simulink model "Child_fuzzy"  (R2023a)
settings: Solver=FixedStepAuto  StartTime=0.0  StopTime=inf  RelTol=1e-3
undefined symbols (not defined in the file): Data_Display, Data_Display1, Data_Display2, Data_Display3, Data_Display4, Data_Display5, Proj
libraries: androiduilib x9, androidaudiovideolib x4, androidcommunicationlib x4, androidsensorlib x3, fuzblock x2
settings Model: Creator=hp  LastModifiedBy=hp
settings OptimizationCC: EnhancedBackFolding=on  PassReuseOutputArgsAs=Individual arguments  ZeroExternalMemoryAtStartup=off  ZeroInternalMemoryAtStartup=off  MaxStackSize=64  OptimizeBlockOrder=speed  DifferentSizesBufferReuse=on  OptimizationCustomize=off  EfficientTunableParamExpr=on
settings DebuggingCC: ParameterTunabilityLossMsg=error
settings HardwareCC: ProdBitPerPointer=32  ProdBitPerSizeT=32  ProdBitPerPtrDiffT=32  ProdLargestAtomicInteger=Long  ProdLargestAtomicFloat=Double  ProdWordSize=32  ProdHWDeviceType=ARM Compatible->ARM Cortex
settings SFSimCC: MATLABDynamicMemAlloc=off
settings RTWCC: Description=Embedded Coder  SystemTargetFile=ert.tlc  HardwareBoard=Android Device  TLCOptions="-aInlineSetEventsForThisBaseRateFcn=TLC_FALSE -aSuppressMultiTaskScheduler=TLC_FALSE  -aRateBasedStepFcn=0"  TemplateMakefile=ert_default_tmf  RTWVerbose=off  Toolchain=Android SDK/NDK Tools
settings CodeAppCC: ForceParamTrailComments=on  IgnoreCustomStorageClasses=off  OperatorAnnotations=on  SimulinkDataObjDesc=on  SFDataObjDesc=on  InsertBlockDesc=on

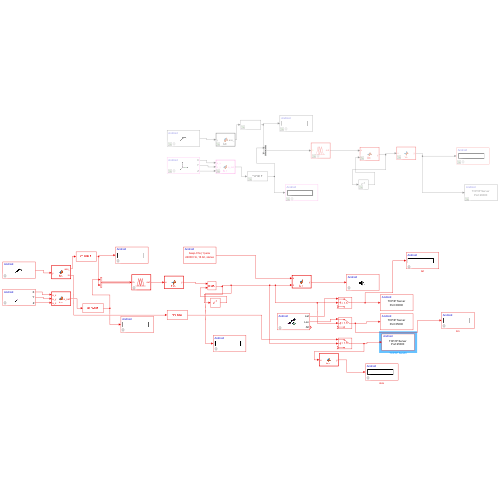
[thumbnail: Simulink's stored preview of the top-level diagram]
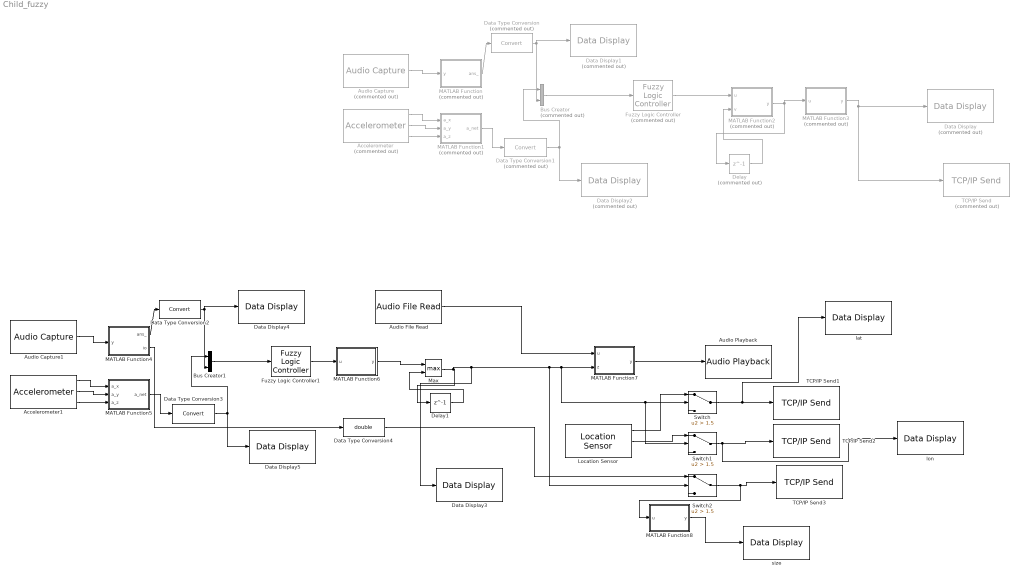
== system Child_fuzzy ==
  Accelerometer : androidsensorlib/Accelerometer  Commented=on  OutputVector=off  SampleTime=0.1  BlockPlatform=Android
  Accelerometer1 : androidsensorlib/Accelerometer  OutputVector=off  SampleTime=0.0125  BlockPlatform=Android
  Audio Capture : androidaudiovideolib/Audio Capture  Commented=on  SampleFreq=8000  FrameSize=4410  SampleTime=0.55125  SimulateUsing=Code generation  DeviceStr=0  QueueDuration=0  BlockPlatform=Android  AudioSamplingFreq=44100
  Audio Capture1 : androidaudiovideolib/Audio Capture  SampleFreq=24000  FrameSize=300  SampleTime=0.0125  SimulateUsing=Code generation  DeviceStr=0  QueueDuration=0  BlockPlatform=Android  AudioSamplingFreq=44100
  Audio File Read : androidaudiovideolib/Audio File Read  FileName=C:\Users\hp\Downloads\beep-01a (1).wav  FrameSize=300
  Audio Playback : androidaudiovideolib/Audio Playback  SampleFreq=24000  AudioSamplingFreq=24000  SampleTime=0.1  DeviceStr=0  QueueDuration=0  BlockPlatform=Android
  Bus Creator : BusCreator  Commented=on  Inputs=2
  Bus Creator1 : BusCreator  Inputs=2
  Data Display : androiduilib/Data Display  Commented=on  DataDisplayId=Proj/Data_Display  Format=Float  Precision=6  SimulateUsing=Code generation  blockPlatform=Android
  Data Display1 : androiduilib/Data Display  Commented=on  DataDisplayId=Proj/Data_Display1  Format=Float  Precision=6  SimulateUsing=Code generation  blockPlatform=Android
  Data Display2 : androiduilib/Data Display  Commented=on  DataDisplayId=Proj/Data_Display2  Format=Float  Precision=6  SimulateUsing=Code generation  blockPlatform=Android
  Data Display3 : androiduilib/Data Display  DataDisplayId=Proj/Data_Display3  Format=Float  Precision=6  SimulateUsing=Code generation  blockPlatform=Android
  Data Display4 : androiduilib/Data Display  DataDisplayId=Proj/Data_Display4  Format=Float  Precision=6  SimulateUsing=Code generation  blockPlatform=Android
  Data Display5 : androiduilib/Data Display  DataDisplayId=Proj/Data_Display5  Format=Float  Precision=6  SimulateUsing=Code generation  blockPlatform=Android
  Data Type Conversion : DataTypeConversion  Commented=on  SaturateOnIntegerOverflow=off  RndMeth=Floor
  Data Type Conversion1 : DataTypeConversion  Commented=on  SaturateOnIntegerOverflow=off  RndMeth=Floor
  Data Type Conversion2 : DataTypeConversion  SaturateOnIntegerOverflow=off  RndMeth=Floor
  Data Type Conversion3 : DataTypeConversion  SaturateOnIntegerOverflow=off  RndMeth=Floor
  Data Type Conversion4 : DataTypeConversion  OutDataTypeStr=double  SaturateOnIntegerOverflow=off  RndMeth=Floor
  Delay : Delay  Commented=on  DelayLength=1  InitialCondition=0
  Delay1 : Delay  DelayLength=1  InitialCondition=0
  Fuzzy Logic Controller : fuzblock/Fuzzy Logic  Controller  Commented=on  FIS='First_Logic.fis'  OutputSampleNumber=101  DataType=double  FuzzifiedInputs=off  RuleFiringStrengths=off  RuleOutputs=off  AggregatedOutputs=off  SimulateUsing=Interpreted execution  OutOfRangeInputValueMessage=warning  NoRuleFiredMessage=warning  EmptyOutputFuzzySetMessage=warning
  Fuzzy Logic Controller1 : fuzblock/Fuzzy Logic  Controller  FIS='First_Logic.fis'  OutputSampleNumber=101  DataType=double  FuzzifiedInputs=off  RuleFiringStrengths=off  RuleOutputs=off  AggregatedOutputs=off  SimulateUsing=Interpreted execution  OutOfRangeInputValueMessage=warning  NoRuleFiredMessage=warning  EmptyOutputFuzzySetMessage=warning
  Location Sensor : androidsensorlib/Location Sensor  OutputVector=off  SampleTime=0.0125  BlockPlatform=Android
  MATLAB Function : MATLAB Function  Commented=on  TreatAsAtomicUnit=on
  MATLAB Function1 : MATLAB Function  Commented=on  TreatAsAtomicUnit=on
  MATLAB Function2 : MATLAB Function  Commented=on  TreatAsAtomicUnit=on
  MATLAB Function3 : MATLAB Function  Commented=on  TreatAsAtomicUnit=on
  MATLAB Function4 : MATLAB Function  TreatAsAtomicUnit=on
  MATLAB Function5 : MATLAB Function  TreatAsAtomicUnit=on
  MATLAB Function6 : MATLAB Function  TreatAsAtomicUnit=on
  MATLAB Function7 : MATLAB Function  TreatAsAtomicUnit=on
  MATLAB Function8 : MATLAB Function  TreatAsAtomicUnit=on
  Max : MinMax  Function=max  Inputs=2
  Switch : Switch  Criteria=u2 > Threshold  Threshold=1.5  SaturateOnIntegerOverflow=off  InputSameDT=off
  Switch1 : Switch  Criteria=u2 > Threshold  Threshold=1.5  SaturateOnIntegerOverflow=off  InputSameDT=off
  Switch2 : Switch  Criteria=u2 > Threshold  Threshold=1.5  SaturateOnIntegerOverflow=off  InputSameDT=off
  TCP/IP Send : androidcommunicationlib/TCP//IP Send  Commented=on  TCPSendId=Proj/TCP//IP_Send  Mode_=Server  LocalServerPort_=26000  RemoteAddr_=127.0.0.1  RemoteServerPort_=25000  ClientPortBindingSelection_=off  ClientPortToBind_=35000  BlockingMode_=off  BlockTimeout_=0.1
  TCP/IP Send1 : androidcommunicationlib/TCP//IP Send  TCPSendId=Proj/TCP//IP_Send1  Mode_=Server  LocalServerPort_=30000  RemoteAddr_=127.0.0.1  RemoteServerPort_=30000  ClientPortBindingSelection_=off  ClientPortToBind_=35000  BlockingMode_=off  BlockTimeout_=0.1
  TCP/IP Send2 : androidcommunicationlib/TCP//IP Send  TCPSendId=Proj/TCP//IP_Send2  Mode_=Server  LocalServerPort_=35000  RemoteAddr_=127.0.0.1  RemoteServerPort_=35000  ClientPortBindingSelection_=off  ClientPortToBind_=35000  BlockingMode_=off  BlockTimeout_=0.1
  TCP/IP Send3 : androidcommunicationlib/TCP//IP Send  TCPSendId=Proj/TCP//IP_Send3  Mode_=Server  LocalServerPort_=25000  RemoteAddr_=127.0.0.1  RemoteServerPort_=25000  ClientPortBindingSelection_=off  ClientPortToBind_=35000  BlockingMode_=off  BlockTimeout_=0.1
  lat : androiduilib/Data Display  DataDisplayId=Proj/lat  Format=Float  Precision=6  SimulateUsing=Code generation  blockPlatform=Android
  lon : androiduilib/Data Display  DataDisplayId=Proj/lon  Format=Float  Precision=6  SimulateUsing=Code generation  blockPlatform=Android
  size : androiduilib/Data Display  DataDisplayId=Proj/size  Format=Float  Precision=6  SimulateUsing=Code generation  blockPlatform=Android
  wires:
  Audio Capture/1 -> MATLAB Function/1(y)
  Bus Creator/1 -> Fuzzy Logic Controller/1
  Accelerometer/1 -> MATLAB Function1/1(a_x)
  Accelerometer/2 -> MATLAB Function1/2(a_y)
  Accelerometer/3 -> MATLAB Function1/3(a_z)
  MATLAB Function/1(ans_) -> Data Type Conversion/1
  Data Type Conversion/1 -> Bus Creator/2, Data Display1/1
  MATLAB Function1/1(a_net) -> Data Type Conversion1/1
  Data Type Conversion1/1 -> Data Display2/1, Bus Creator/1
  MATLAB Function2/1(y) -> MATLAB Function3/1(u), Delay/1
  Delay/1 -> MATLAB Function2/2(v)
  MATLAB Function3/1(y) -> Data Display/1, TCP/IP Send/1
  Fuzzy Logic Controller/1 -> MATLAB Function2/1(u)
  Data Type Conversion3/1 -> Data Display5/1, Bus Creator1/1
  MATLAB Function4/1(ans_) -> Data Type Conversion2/1
  Data Type Conversion2/1 -> Bus Creator1/2, Data Display4/1
  Accelerometer1/2 -> MATLAB Function5/2(a_y)
  Audio Capture1/1 -> MATLAB Function4/1(y)
  MATLAB Function5/1(a_net) -> Data Type Conversion3/1
  Accelerometer1/1 -> MATLAB Function5/1(a_x)
  Accelerometer1/3 -> MATLAB Function5/3(a_z)
  Bus Creator1/1 -> Fuzzy Logic Controller1/1
  Fuzzy Logic Controller1/1 -> MATLAB Function6/1(u)
  MATLAB Function7/1(y) -> Audio Playback/1
  Audio File Read/1 -> MATLAB Function7/1(u)
  MATLAB Function6/1(y) -> Max/1
  Max/1 -> Data Display3/1, Switch2/2, Switch1/2, Switch/2, MATLAB Function7/2(z), Delay1/1
  Delay1/1 -> Max/2
  Switch/1 -> lat/1, TCP/IP Send1/1
  Location Sensor/1 -> Switch/1
  Location Sensor/2 -> Switch1/1
  Switch1/1 -> lon/1, TCP/IP Send2/1
  Switch2/1 -> MATLAB Function8/1(u), TCP/IP Send3/1
  MATLAB Function4/2(io) -> Data Type Conversion4/1
  MATLAB Function8/1(y) -> size/1
  Data Type Conversion4/1 -> Switch2/1

== matlab function Child_fuzzy/MATLAB Function1 ==
  data: a_x input; a_net output; a_y input; a_z input
function a_net = fcn(a_x,a_y,a_z)

a_net = (a_x ^ 2 + a_y ^ 2 + a_z ^ 2) ^ 0.5 ;

== matlab function Child_fuzzy/MATLAB Function ==
  data: y input; ans_ output
function ans_ = fcn(y)
    
left_channel = max(y(:, 1));
right_channel = max(y(:, 2));

% if max(left_channel,right_channel) > 28000 
%     ans_ = 20 ;
% elseif max(left_channel,right_channel) > 15000 
%     ans_ = 10 ;
% else 
%     ans_ = 0 ;

ans_ = max(left_channel,right_channel);
end

== matlab function Child_fuzzy/MATLAB Function2 ==
  data: u input; y output; v input
function y = fcn(u,v)

z = max(u,v);
if (z > 0.5) 
    y = z ;
else 
    y = u ;
end 
% 
% function y = fcn(v)
% persistent flag;
% 
%     if isempty(flag)
%         flag = 0;
%     end
%     if v > 0.70
%         flag = 2;
%         y = 2;
%     elseif v > 0.35
%         flag = 1;
%         y = 1;
%     else
%         flag = 0;
%         y = 0;
%     end
% end

== matlab function Child_fuzzy/MATLAB Function3 ==
  data: u input; y output
function y = fcn(u)
    if u <= 0.35 
        y = 0 ; 
    elseif u <= 0.7 
        y = 1 ; 
    else
        y = 2 ; 
    end

== matlab function Child_fuzzy/MATLAB Function4 ==
  data: y input; ans_ output; io output
function [ans_,io] = fcn(y)
    
ans_ = max(y(:, 1));
io = y(:, 1) ;
%right_channel = max(y(:, 2));

% if max(left_channel,right_channel) > 28000 
%     ans_ = 20 ;
% elseif max(left_channel,right_channel) > 15000 
%     ans_ = 10 ;
% else 
%     ans_ = 0 ;

%ans_ = max(left_channel,right_channel);
end

== matlab function Child_fuzzy/MATLAB Function5 ==
  data: a_x input; a_net output; a_y input; a_z input
function a_net = fcn(a_x,a_y,a_z)

a_net = (a_x ^ 2 + a_y ^ 2 + a_z ^ 2) ^ 0.5 ;

== matlab function Child_fuzzy/MATLAB Function6 ==
  data: u input; y output
function y = fcn(u)

if (u > 0.7)
    y = 2 ; 
elseif (u > 0.35)
    y = 1 ; 
else 
    y = 0 ; 
end

== matlab function Child_fuzzy/MATLAB Function7 ==
  data: u input; z input; y output
function y = fcn(u,z)
    if z == 1
        % Convert u to int16 before concatenation
        
        y = u; 
    elseif z == 2
        % Convert the first 31542 elements of v to int16
        u = u * 200000 ;
        
        y = u;         
    else 
        % Return a 2-channel array of zeros based on u
        y = zeros(size(u, 1), 2, 'int16');
    end
end

== matlab function Child_fuzzy/MATLAB Function8 ==
  data: u input; y output
function y = fcn(u)

y = size(u);
